simulink model "DC_Motor_And_Chasis_Dynamic_Model"  (R2020b)
settings: Solver=VariableStepAuto  StartTime=0.0  StopTime=50  RelTol=1e-3
values from neighbouring files (symbols this model uses):
  a = 0    [Robot_Parameters.m]
  b = 0.2    [Robot_Parameters.m]
  I = 0.08    [Robot_Parameters.m]
  Ke = 0.03    [Robot_Parameters.m]
  Kt = 0.001    [Robot_Parameters.m]
  L = 0.01    [Robot_Parameters.m]
  m = 1.733    [Robot_Parameters.m]
  N = 30    [Robot_Parameters.m]
  r = 0.0425    [Robot_Parameters.m]
  R = 0.7    [Robot_Parameters.m]
settings Model: OrderedModelArguments=off  Creator=dell  LastModifiedBy=dell

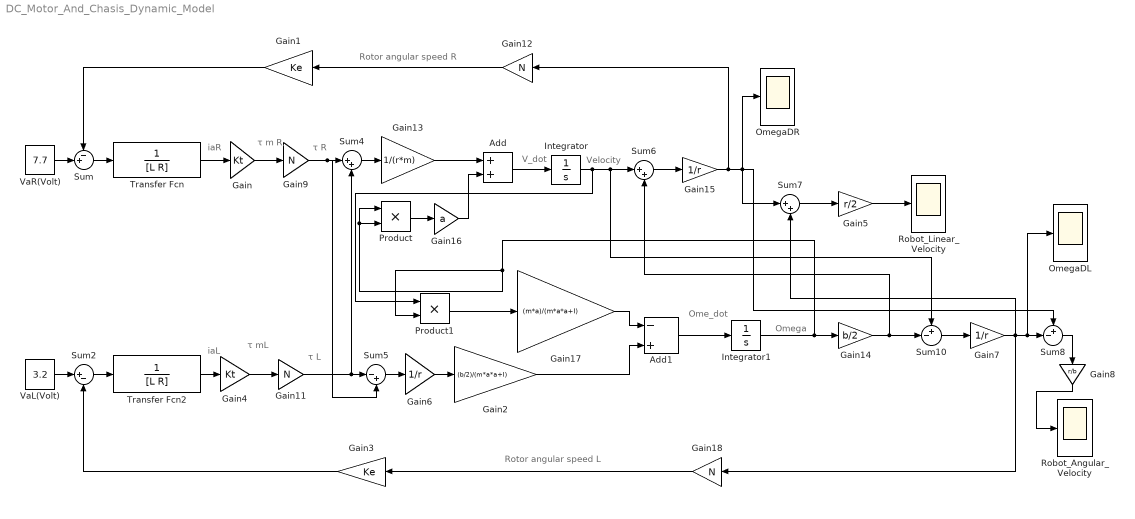
== system DC_Motor_And_Chasis_Dynamic_Model ==
  note: Rotor angular speed R
  note: Velocity
  note: V_dot
  note: Omega
  note: Ome_dot
  note: τ R
  note: τ m R
  note: iaR
  note: iaL
  note: τ mL
  note: τ L
  note: Rotor angular speed L
  Add : Sum
  Add1 : Sum  Inputs=-+
  Gain : Gain  Gain=Kt
  Gain1 : Gain  Gain=Ke
  Gain{9,11..12,18} (4 alike) : Gain  Gain=N
  Gain13 : Gain  Gain=1/(r*m)
  Gain14 : Gain  Gain=b/2
  Gain15 : Gain  Gain=1/r
  Gain16 : Gain  Gain=a
  Gain17 : Gain  Gain=(m*a)/(m*a*a+I)
  Gain2 : Gain  Gain=(b/2)/(m*a*a+I)
  Gain3 : Gain  Gain=Ke
  Gain4 : Gain  Gain=Kt
  Gain5 : Gain  Gain=r/2
  Gain6 : Gain  Gain=1/r
  Gain7 : Gain  Gain=1/r
  Gain8 : Gain  Gain=r/b
  Integrator : Integrator
  Integrator1 : Integrator
  OmegaDL : Scope
  OmegaDR : Scope
  Product : Product
  Product1 : Product
  Robot_Angular_Velocity : Scope
  Robot_Linear_Velocity : Scope
  Sum : Sum  Inputs=-+|
  Sum10 : Sum  Inputs=+-|
  Sum2 : Sum  Inputs=|+-
  Sum4 : Sum  Inputs=|++
  Sum5 : Sum  Inputs=|-+
  Sum6 : Sum  Inputs=|++
  Sum7 : Sum  Inputs=|++
  Sum8 : Sum  Inputs=+-|
  Transfer Fcn : TransferFcn  Denominator=[L R]
  Transfer Fcn2 : TransferFcn  Denominator=[L R]
  VaL(Volt) : Constant  Value=3.2
  VaR(Volt) : Constant  Value=7.7
  wires:
  Gain3/1 -> Sum2/2
  Sum4/1 -> Gain13/1
  Transfer Fcn2/1 -> Gain4/1
  Transfer Fcn/1 -> Gain/1
  Gain/1 -> Gain9/1
  Gain9/1 -> Sum4/1, Sum5/2
  Gain4/1 -> Gain11/1
  Gain11/1 -> Sum5/1, Sum4/2
  Gain13/1 -> Add/1
  Sum5/1 -> Gain6/1
  Gain6/1 -> Gain2/1
  Gain2/1 -> Add1/2
  Add1/1 -> Integrator1/1
  Integrator1/1 -> Gain14/1, Product/2, Product/1, Product1/2
  Add/1 -> Integrator/1
  Sum6/1 -> Gain15/1
  Integrator/1 -> Sum6/1, Sum10/1, Product1/1
  Gain14/1 -> Sum10/2, Sum6/2
  Sum10/1 -> Gain7/1
  Product/1 -> Gain16/1
  Product1/1 -> Gain17/1
  Gain15/1 -> Sum8/1, Sum7/1, OmegaDR/1, Gain12/1
  Gain7/1 -> Sum8/2, OmegaDL/1, Sum7/2, Gain18/1
  Sum7/1 -> Gain5/1
  Gain5/1 -> Robot_Linear_Velocity/1
  Sum8/1 -> Gain8/1
  Gain8/1 -> Robot_Angular_Velocity/1
  Gain16/1 -> Add/2
  Gain17/1 -> Add1/1
  Sum/1 -> Transfer Fcn/1
  Sum2/1 -> Transfer Fcn2/1
  VaL(Volt)/1 -> Sum2/1
  Gain18/1 -> Gain3/1
  VaR(Volt)/1 -> Sum/2
  Gain1/1 -> Sum/1
  Gain12/1 -> Gain1/1
